simulink model "quad_model"  (R2015b)
settings: Solver=VariableStepAuto  StartTime=0.0  StopTime=100  RelTol=1e-3
undefined symbols (not defined in the file): IX, IY, IZ, Jr, L, M
settings Model: Creator=root  LastModifiedBy=root

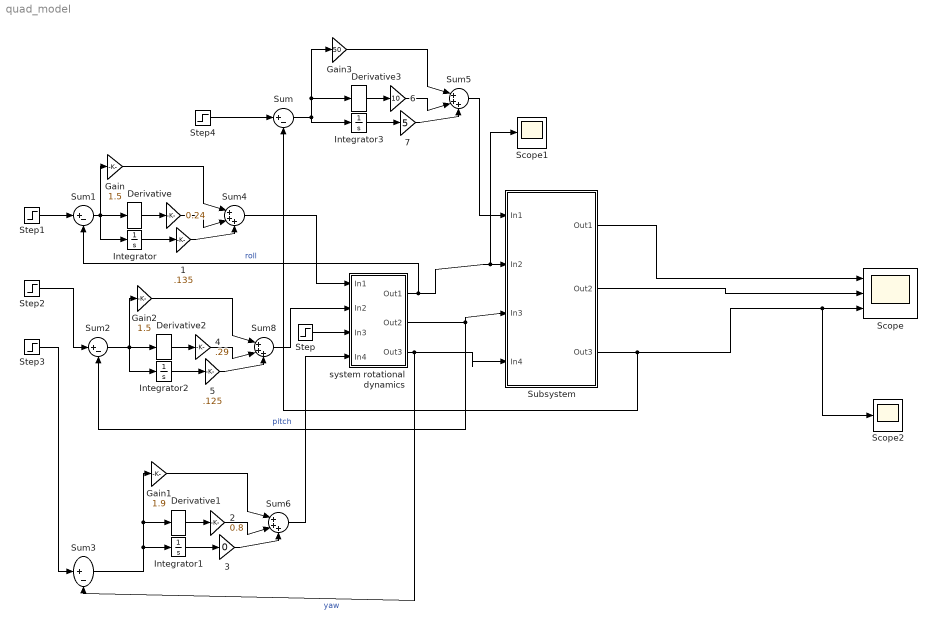
== system quad_model ==
  " " : Gain  Gain=0.24
  " 1" : Gain  Gain=.135
  " 2" : Gain  Gain=0.8
  " 3" : Gain  Gain=0
  " 4" : Gain  Gain=.29
  " 5" : Gain  Gain=.125
  " 6" : Gain  Gain=10
  " 7" : Gain  Gain=5
  Derivative{,1..3} (4 alike) : Derivative
  Gain : Gain  Gain=1.5
  Gain1 : Gain  Gain=1.9
  Gain2 : Gain  Gain=1.5
  Gain3 : Gain  Gain=50
  Integrator{,1..3} (4 alike) : Integrator
  Scope : Scope  NumInputPorts=3
  Scope1 : Scope
  Scope2 : Scope
  Step : Step  Time=0  After=0  SampleTime=0
  Step1 : Step  Time=0  After=0.261667  SampleTime=0
  Step2 : Step  Time=0  After=0.0349065  SampleTime=0
  Step3 : Step  Time=0  After=0  SampleTime=0
  Step4 : Step  Time=0  After=5  SampleTime=0
  Subsystem : Subsystem
  Sum{,1..3} (4 alike) : Sum  Inputs=|+-
  Sum{4..6,8} (4 alike) : Sum  Inputs=|+++
  system rotational dynamics : Subsystem
  wires:
  system rotational dynamics/1(Out1) -> Scope1/1, Subsystem/2(In2), Sum1/2  "roll"
  system rotational dynamics/2(Out2) -> Subsystem/3(In3), Sum2/2  "pitch"
  system rotational dynamics/3(Out3) -> Subsystem/4(In4), Sum3/2  "yaw"
  Subsystem/1(Out1) -> Scope/1
  Subsystem/2(Out2) -> Scope/2
  Subsystem/3(Out3) -> Sum/2, Scope2/1, Scope/3
  Step/1 -> system rotational dynamics/3(In3)
  Step2/1 -> Sum2/1
  Step3/1 -> Sum3/1
  Step1/1 -> Sum1/1
  Step4/1 -> Sum/1
  Derivative/1 -> " "/1
  Gain/1 -> Sum4/1
  " "/1 -> Sum4/2
  Sum1/1 -> Integrator/1, Derivative/1, Gain/1
  Integrator/1 -> " 1"/1
  " 1"/1 -> Sum4/3
  Sum4/1 -> system rotational dynamics/1(In1)
  Derivative1/1 -> " 2"/1
  Gain1/1 -> Sum6/1
  " 2"/1 -> Sum6/2
  Sum3/1 -> Derivative1/1, Gain1/1, Integrator1/1
  Integrator1/1 -> " 3"/1
  " 3"/1 -> Sum6/3
  Derivative2/1 -> " 4"/1
  Gain2/1 -> Sum8/1
  " 4"/1 -> Sum8/2
  Sum2/1 -> Integrator2/1, Derivative2/1, Gain2/1
  Integrator2/1 -> " 5"/1
  " 5"/1 -> Sum8/3
  Sum6/1 -> system rotational dynamics/4(In4)
  Sum8/1 -> system rotational dynamics/2(In2)
  Derivative3/1 -> " 6"/1
  Gain3/1 -> Sum5/1
  " 6"/1 -> Sum5/2
  Integrator3/1 -> " 7"/1
  " 7"/1 -> Sum5/3
  Sum/1 -> Derivative3/1, Gain3/1, Integrator3/1
  Sum5/1 -> Subsystem/1(In1)

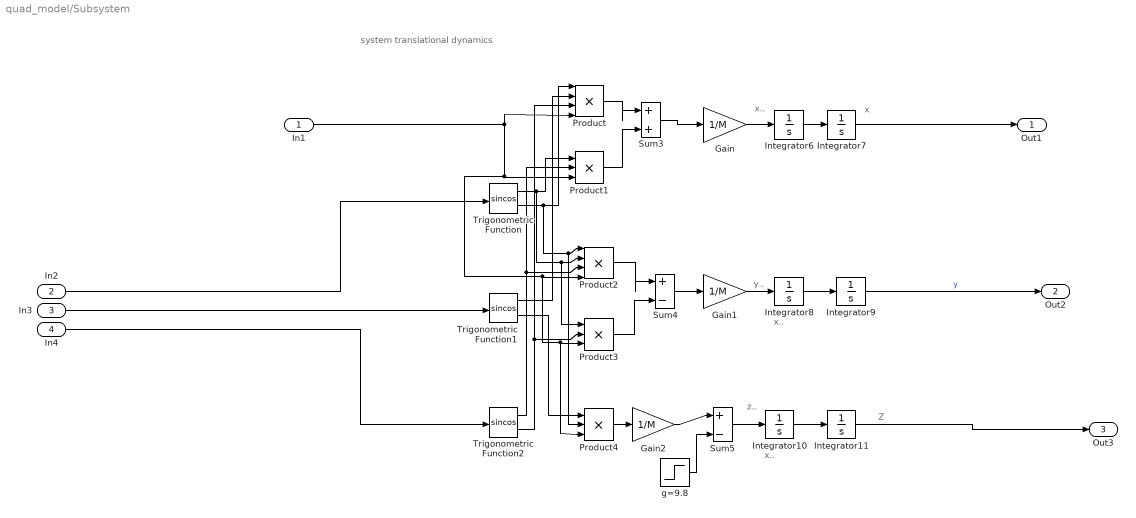
== system quad_model/Subsystem ==
  note: system translational dynamics
  note: x..
  note: x..
  note: x..
  note: x
  note: y..
  note: Z
  note: z..
  In1 : Inport
  In2 : Inport  Port=2
  In3 : Inport  Port=3
  In4 : Inport  Port=4
  Gain : Gain  Gain=1/M
  Gain1 : Gain  Gain=1/M
  Gain2 : Gain  Gain=1/M
  Integrator{8..11} (4 alike) : Integrator
  Integrator6 : Integrator  InitialCondition=0.0
  Integrator7 : Integrator  InitialCondition=0.0
  Product : Product  Inputs=4
  Product1 : Product  Inputs=3
  Product2 : Product  Inputs=4
  Product3 : Product  Inputs=3
  Product4 : Product  Inputs=3
  Sum3 : Sum  Inputs=|++
  Sum4 : Sum  Inputs=|+-
  Sum5 : Sum  Inputs=|+-
  Trigonometric Function : Trigonometry  Operator=sincos
  Trigonometric Function1 : Trigonometry  Operator=sincos
  Trigonometric Function2 : Trigonometry  Operator=sincos
  g=9.8 : Step  Time=0  After=9.81  SampleTime=0
  Out1 : Outport
  Out2 : Outport  Port=2
  Out3 : Outport  Port=3
  wires:
  In1/1 -> Product/4, Product1/3, Product4/3, Product3/3, Product2/4
  Integrator8/1 -> Integrator9/1
  Trigonometric Function1/2 -> Product4/1
  Integrator6/1 -> Integrator7/1
  Product3/1 -> Sum4/2
  Product4/1 -> Gain2/1
  Gain1/1 -> Integrator8/1
  Integrator10/1 -> Integrator11/1
  Gain2/1 -> Sum5/1
  Sum5/1 -> Integrator10/1
  g=9.8/1 -> Sum5/2
  Sum3/1 -> Gain/1
  Trigonometric Function/2 -> Product4/2, Product2/1, Product/1
  Integrator7/1 -> Out1/1
  Product1/1 -> Sum3/2
  Product/1 -> Sum3/1
  Trigonometric Function1/1 -> Product/2
  Trigonometric Function/1 -> Product1/1, Product3/1, Product2/2
  Trigonometric Function2/1 -> Product2/3, Product1/2
  Product2/1 -> Sum4/1
  Sum4/1 -> Gain1/1
  Gain/1 -> Integrator6/1
  Trigonometric Function2/2 -> Product3/2, Product/3
  Integrator9/1 -> Out2/1  "y"
  Integrator11/1 -> Out3/1
  In2/1 -> Trigonometric Function/1
  In3/1 -> Trigonometric Function1/1
  In4/1 -> Trigonometric Function2/1

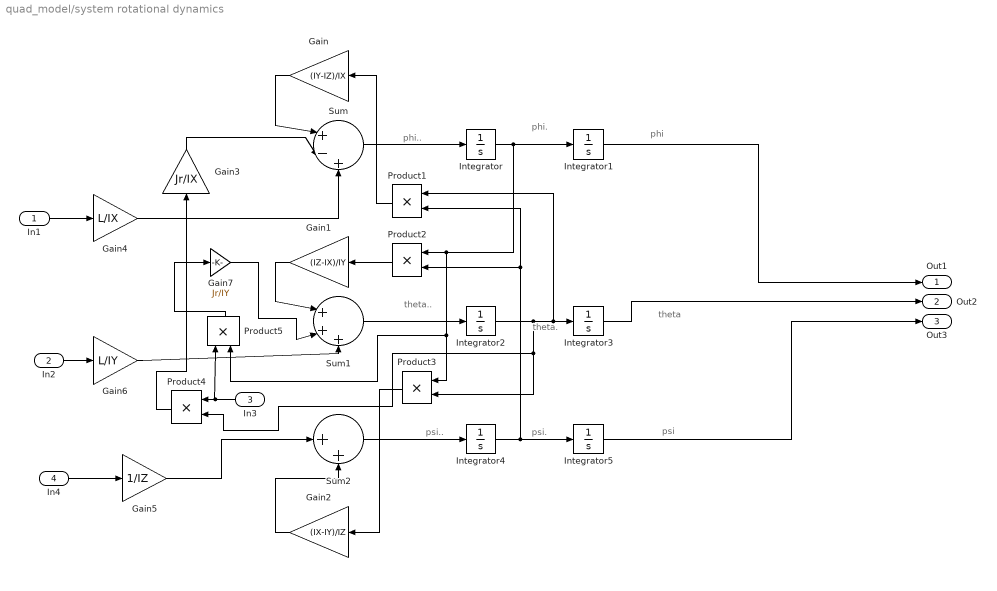
== system quad_model/system rotational dynamics ==
  note: psi
  note: theta
  note: phi
  note: psi.
  note: psi..
  note: theta.
  note: theta..
  note: phi.
  note: phi..
  In1 : Inport
  In2 : Inport  Port=2
  In3 : Inport  Port=3
  In4 : Inport  Port=4
  Gain : Gain  Gain=(IY-IZ)/IX
  Gain1 : Gain  Gain=(IZ-IX)/IY
  Gain2 : Gain  Gain=(IX-IY)/IZ
  Gain3 : Gain  Gain=Jr/IX
  Gain4 : Gain  Gain=L/IX
  Gain5 : Gain  Gain=1/IZ
  Gain6 : Gain  Gain=L/IY
  Gain7 : Gain  Gain=Jr/IY
  Integrator{,1..5} (6 alike) : Integrator  InitialCondition=0.0
  Product{1..5} (5 alike) : Product
  Sum : Sum  Inputs=|+-+
  Sum1 : Sum  Inputs=|+++
  Sum2 : Sum  Inputs=|++
  Out1 : Outport
  Out2 : Outport  Port=2
  Out3 : Outport  Port=3
  wires:
  Gain4/1 -> Sum/3
  Product2/1 -> Gain1/1
  Gain5/1 -> Sum2/1
  Gain2/1 -> Sum2/2
  Gain6/1 -> Sum1/3
  In2/1 -> Gain6/1
  Integrator3/1 -> Out2/1
  Gain1/1 -> Sum1/1
  Integrator1/1 -> Out1/1
  Integrator5/1 -> Out3/1
  Product4/1 -> Gain3/1
  Product1/1 -> Gain/1
  Gain/1 -> Sum/1
  In3/1 -> Product5/1, Product4/1
  Gain3/1 -> Sum/2
  Product5/1 -> Gain7/1
  Gain7/1 -> Sum1/2
  Sum2/1 -> Integrator4/1
  Sum1/1 -> Integrator2/1
  Product3/1 -> Gain2/1
  In4/1 -> Gain5/1
  In1/1 -> Gain4/1
  Integrator/1 -> Product5/2, Product3/1, Product2/1, Integrator1/1
  Integrator2/1 -> Product4/2, Product3/2, Product1/1, Integrator3/1
  Integrator4/1 -> Product2/2, Product1/2, Integrator5/1
  Sum/1 -> Integrator/1
